simulink model "spielwiese"  (Simulink 6.5)
settings: Solver=FixedStepDiscrete  StartTime=0.0  StopTime=inf  RelTol=1e-3
settings Model: Creator=sja  LastModifiedBy=sja  ExtModeAutoUpdateStatusClock=off
settings DebuggingCC: MultiTaskDSMMsg=warning  MultiTaskCondExecSysMsg=none  StrictBusMsg=None
settings RTWCC: IncludeERTFirstTime=on

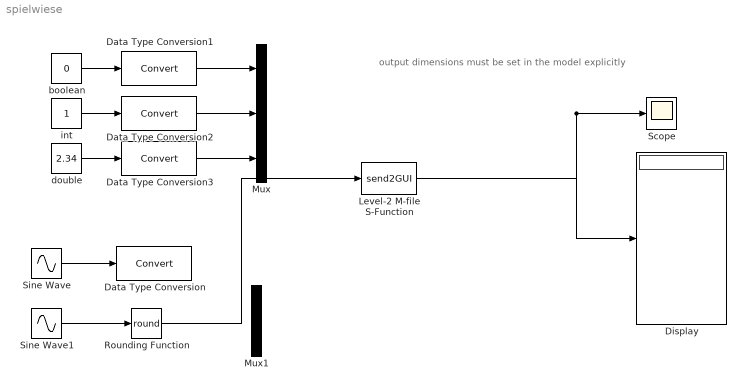
== system spielwiese ==
  note: output dimensions must
      | be set in the model
      | explicitly
  Data Type Conversion : DataTypeConversion  OutDataTypeMode=int16
  Data Type Conversion1 : DataTypeConversion
  Data Type Conversion2 : DataTypeConversion
  Data Type Conversion3 : DataTypeConversion
  Display : Display
  Level-2 M-file S-Function : M-S-Function  FunctionName=send2GUI  mask{sampletime=0}
  Mux : Mux  Inputs=3
  Mux1 : Mux
  Rounding Function : Rounding  Operator=round
  Scope : Scope
      settings: YMin=0.95  YMax=1.05
  Sine Wave : Sin  Bias=1  Frequency=2  Phase=100  Samples=100  SampleTime=0.0001
  Sine Wave1 : Sin  Amplitude=50  Bias=1  Frequency=2  Phase=100  Samples=100  SampleTime=0.0001
  boolean : Constant  Value=0  OutDataTypeMode=boolean  OutDataType=sfix(16)  ConRadixGroup=Use specified scaling  OutScaling=2^0  SampleTime=inf  FramePeriod=inf
  double : Constant  Value=2.34  OutDataTypeMode=double  OutDataType=sfix(16)  ConRadixGroup=Use specified scaling  OutScaling=2^0  SampleTime=inf  FramePeriod=inf
  int : Constant  Value=1  OutDataTypeMode=int32  OutDataType=sfix(16)  ConRadixGroup=Use specified scaling  OutScaling=2^0  SampleTime=inf  FramePeriod=inf
  wires:
  Sine Wave/1 -> Data Type Conversion/1
  Level-2 M-file S-Function/1 -> Scope/1, Display/1
  boolean/1 -> Data Type Conversion1/1
  int/1 -> Data Type Conversion2/1
  double/1 -> Data Type Conversion3/1
  Data Type Conversion1/1 -> Mux/1
  Data Type Conversion2/1 -> Mux/2
  Data Type Conversion3/1 -> Mux/3
  Sine Wave1/1 -> Rounding Function/1
  Rounding Function/1 -> Level-2 M-file S-Function/1
